simulink model "ps1m"  (R2013b)
settings: Solver=ode45  StartTime=0.0  StopTime=10.0  RelTol=1e-3
libraries: fl_lib x17, nesl_utility x5
settings Model: Creator=xmax1946  LastModifiedBy=xmax1946

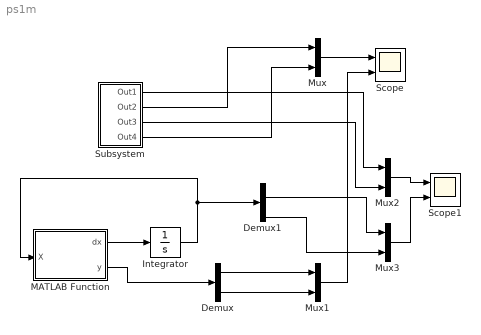
== system ps1m ==
  Demux : Demux  Outputs=2
  Demux1 : Demux
  Integrator : Integrator  InitialCondition=[0;0;0;0]
  MATLAB Function : MATLAB Function  TreatAsAtomicUnit=on
  Mux{,1..3} (4 alike) : Mux  Inputs=2
  Scope : Scope  NumInputPorts=2
      settings: YMin=-5~-5  YMax=5~5
  Scope1 : Scope  NumInputPorts=2
      settings: YMin=-5~-5  YMax=5~5
  Subsystem : Subsystem
  wires:
  MATLAB Function/1(dx) -> Integrator/1
  Integrator/1 -> Demux1/1, MATLAB Function/1(X)
  MATLAB Function/2(y) -> Demux/1
  Subsystem/2(Out2) -> Mux/1
  Mux1/1 -> Scope/2
  Mux/1 -> Scope/1
  Subsystem/4(Out4) -> Mux/2
  Demux/1 -> Mux1/1
  Demux/2 -> Mux1/2
  Subsystem/1(Out1) -> Mux2/1
  Demux1/4 -> Mux3/2
  Mux2/1 -> Scope1/1
  Mux3/1 -> Scope1/2
  Subsystem/3(Out3) -> Mux2/2
  Demux1/2 -> Mux3/1

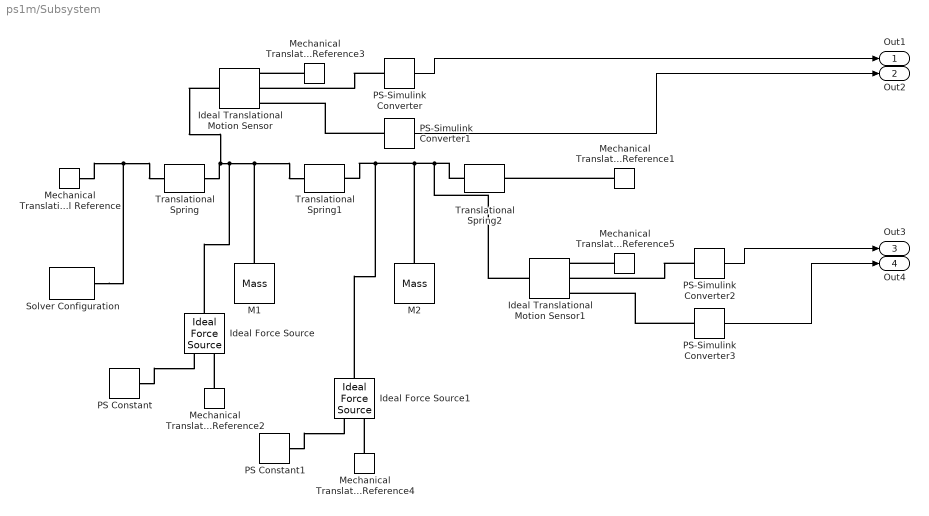
== system ps1m/Subsystem ==
  Ideal Force Source : fl_lib/Mechanical/Mechanical Sources/Ideal Force Source  v_Log=off  f_Log=off  LocalVarNames=|v|f  LocalVarDescs=|v|f  LocalVarLogging=[0 0]
  Ideal Force Source1 : fl_lib/Mechanical/Mechanical Sources/Ideal Force Source  v_Log=off  f_Log=off  LocalVarNames=|v|f  LocalVarDescs=|v|f  LocalVarLogging=[0 0]
  Ideal Translational Motion Sensor : fl_lib/Mechanical/Mechanical Sensors/Ideal Translational Motion Sensor  offset=0 m  v_Log=off  f_Log=off  x_Log=off  LocalVarNames=|v|f|x  LocalVarDescs=|v|f|x  LocalVarLogging=[0 0 0]
  Ideal Translational Motion Sensor1 : fl_lib/Mechanical/Mechanical Sensors/Ideal Translational Motion Sensor  offset=0 m  v_Log=off  f_Log=off  x_Log=off  LocalVarNames=|v|f|x  LocalVarDescs=|v|f|x  LocalVarLogging=[0 0 0]
  M1 : fl_lib/Mechanical/Translational Elements/Mass  mass=3 kg  initial_velocity=0 m/s  f_Log=off  LocalVarNames=|f  LocalVarDescs=|f  LocalVarLogging=0
  M2 : fl_lib/Mechanical/Translational Elements/Mass  mass=1 kg  initial_velocity=0 m/s  f_Log=off  LocalVarNames=|f  LocalVarDescs=|f  LocalVarLogging=0
  Mechanical Translational Reference{,1..5} (6 alike) : fl_lib/Mechanical/Translational Elements/Mechanical Translational Reference  f_Log=off  LocalVarNames=|f  LocalVarDescs=|f  LocalVarLogging=0
  PS Constant : fl_lib/Physical Signals/Sources/PS Constant  constant=10  LocalVarLogging=[]
  PS Constant1 : fl_lib/Physical Signals/Sources/PS Constant  constant=8  LocalVarLogging=[]
  PS-Simulink Converter{,1..3} (4 alike) : nesl_utility/PS-Simulink Converter  PhysicalDomain=network_engine_domain  SubClassName=ps_output  LeftPortType=input  RightPortType=output  PseudoPeriodic=off  Frequencies=[]  Unit=1  AffineConversion=off
  Solver Configuration : nesl_utility/Solver Configuration  PhysicalDomain=network_engine_domain  SubClassName=solver  LeftPortType=input  RightPortType=generic  Accelerate=off  Tones=[]  Harmonics=[]  SimulateNoise=off  Profile=off  UseLocalSampling=off  EnableSwitchedLinearOptims=on  FrequencyDomain=off  UseCCode=off  RelTol=0.001  AbsTol=1e-06  MinStep=1e-09  ToWorkspace=off  DoDC=off  ResidualTolerance=1e-09  UseLocalSolver=off  LocalSolverChoice=NE_BACKWARD_EULER_ADVANCER  LocalSolverSampleTime=0.001  DoFixedCost=off  MaxNonlinIter=3  MaxModeIter=2  LinearAlgebra=Sparse  DelaysMemoryBudget=1024
  Translational Spring : fl_lib/Mechanical/Translational Elements/Translational Spring  spr_rate=10 N/m  init_def=0 m  f_Log=off  v_Log=off  x_Log=off  LocalVarNames=|f|v|x  LocalVarDescs=|f|v|x  LocalVarLogging=[0 0 0]
  Translational Spring1 : fl_lib/Mechanical/Translational Elements/Translational Spring  spr_rate=8 N/m  init_def=0 m  f_Log=off  v_Log=off  x_Log=off  LocalVarNames=|f|v|x  LocalVarDescs=|f|v|x  LocalVarLogging=[0 0 0]
  Translational Spring2 : fl_lib/Mechanical/Translational Elements/Translational Spring  spr_rate=10 N/m  init_def=0 m  f_Log=off  v_Log=off  x_Log=off  LocalVarNames=|f|v|x  LocalVarDescs=|f|v|x  LocalVarLogging=[0 0 0]
  Out1 : Outport
  Out2 : Outport  Port=2
  Out3 : Outport  Port=3
  Out4 : Outport  Port=4
  wires:
  PS-Simulink Converter2/1 -> Out3/1
  PS-Simulink Converter1/1 -> Out2/1
  PS-Simulink Converter3/1 -> Out4/1
  PS-Simulink Converter/1 -> Out1/1
  connections:
  Mechanical Translational Reference/LConn1 -- Solver Configuration/RConn1 -- Translational Spring/LConn1
  PS Constant1/RConn1 -- Ideal Force Source1/RConn1
  Mechanical Translational Reference4/LConn1 -- Ideal Force Source1/RConn2
  PS-Simulink Converter/LConn1 -- Ideal Translational Motion Sensor/RConn2
  Mechanical Translational Reference3/LConn1 -- Ideal Translational Motion Sensor/RConn1
  Translational Spring/RConn1 -- Ideal Translational Motion Sensor/LConn1 -- M1/LConn1 -- Translational Spring1/LConn1 -- Ideal Force Source/LConn1
  Mechanical Translational Reference2/LConn1 -- Ideal Force Source/RConn2
  PS Constant/RConn1 -- Ideal Force Source/RConn1
  Translational Spring2/LConn1 -- Ideal Translational Motion Sensor1/LConn1 -- M2/LConn1 -- Ideal Force Source1/LConn1 -- Translational Spring1/RConn1
  Mechanical Translational Reference1/LConn1 -- Translational Spring2/RConn1
  PS-Simulink Converter1/LConn1 -- Ideal Translational Motion Sensor/RConn3
  Mechanical Translational Reference5/LConn1 -- Ideal Translational Motion Sensor1/RConn1
  PS-Simulink Converter3/LConn1 -- Ideal Translational Motion Sensor1/RConn3
  PS-Simulink Converter2/LConn1 -- Ideal Translational Motion Sensor1/RConn2

== matlab function ps1m/MATLAB Function ==
  data: dx output; X input; y output
function [dx,y] = fcn(X)
m1=3;
m2=1;
k1=10;
k2=8;
u1=10;
u2=8;
A=[0,1,0,0;-(k1+k2)/m1,0,k2/m1,0;0,0,0,1;k2/m2,0,-(k1+k2)/m2,0];
B=[0,0;1/m1,0;0,0;0,1/m2];
C=[1,0,0,0;0,0,1,0];
U=[u1;u2];
dx=A*X+B*U;
y=C*X;
